simulink model "VirtualVehicleTemplate"  (R2023a)
settings: configuration reference "VehicleVariable" (kept outside this file)
StartFcn:
  | %tic
StopFcn:
  | %toc
undefined symbols (not defined in the file): CtrlEcuRevLim, CtrlTcuInitGear, CtrlVcuCltch1InitCmd, Disabled, DriverPreviewDist, EnvAbsPrs, EnvAirTemp, EnvGrvty, EnvNomFrictionScaling, EnvNominalGrade, EnvWindVelX, EnvWindVelY, EnvWindVelZ, FTP75, PlntVehDstCGFrntAxl, PlntVehDstCGRearAxl, PlntVehInitLatPos, PlntVehInitLongPos, PlntVehInitPitchAng, PlntVehInitRollAng, PlntVehInitVertPos, PlntVehInitYawAng, PlntVehMass, PlntVehTrckWdth, PlntVehYawMomentInertia, ScnCRMaxLatAccel, ScnCRRadius, ScnDLCGateLongPos, ScnDLCLatRef, ScnDLCLatRefOffset, ScnDLCLongRefBpt, ScnDLCLongRefStartPos, ScnDLCVehicleWidth, ScnFHCounterDwellTime, ScnFHInitialDwellTime, ScnFHReturnTime, ScnFHRollRateZeroCross, ScnFHSteerAmp, ScnFHSteerSpeed, ScnISHandwheelRate, ScnISMaxHandwheelAng, ScnISMaxLatAccel, ScnISSteerHoldTime, ScnLongVelRef, ScnSDDwellTime, ScnSDSteerAmp, ScnSDSteerFreq, ScnSimTime, ScnSSFinalFreq, ScnSSSteerAmp, ScnSSSweepTime, ScnStartTime
libraries: simulink x18, vehdynlibscenariocommon x7, vehdynlibviscommon x3, vehdynlibdriver x2, sim3dgroundtruthsensorlib x2, autolibshared x2, autolibsharedcommon x1, sharedtransform x1, sim3dlib x1, sim3dautolib x1
(part 5 of 5)

== system VirtualVehicleTemplate/Environment/Ground Feedback/3D Engine/3D Engine Source/Single Point ==
  Bus Creator1 : BusCreator  Inputs=4
  Bus Selector2 : BusSelector  OutputSignals=Wheel1Positions,Wheel2Positions,Wheel3Positions,Wheel4Positions
  Constant2 : Constant  Value=repmat(eye(3),1,1,4)  SampleTime=-1
  Data Type Conversion{1..4} (4 alike) : DataTypeConversion  SaturateOnIntegerOverflow=off  RndMeth=Floor
  First Order Hold{5..8} (4 alike) : FirstOrderHold  ErrorTolerance=1
  Range Limiter{5..8} (4 alike) : Saturate  UpperLimit=1e3  LowerLimit=-1e3  ZeroCross=off
  Signal Specification{6..9} (4 alike) : SignalSpecification  Unit=m
  Simulation 3D Terrain Sensor1 : sim3dgroundtruthsensorlib/Simulation 3D Terrain Sensor  Priority=1  sensorTag=Sim3dSensor1  sensorId=1  sensorName=Sim3dSensor1  VehicleIdentifier=SimulinkVehicle1  tmountOffset=[0, 0, 0]  rmountOffset=[0,0,0,]  RayOrigins=[0 0 1]  RayDirections=[0 0 -1]  RayLengths=20  NumberOfWheels=4  VisualizeTraceLines=off  SampleTime=-1  aMode=2  ID=1
  Zend Select{1..4} (4 alike) : Selector  NumberOfDimensions=2  InputPortWidth=3  IndexOptions=Select all,Index vector (dialog)  Indices=[1 3],3  OutputSizes=1,1
  z : Outport
  DCM : Outport  Port=2
  wires:
  Signal Specification6/1 -> Bus Creator1/1  "G_FL_z"
  Simulation 3D Terrain Sensor1/1 -> Bus Selector2/1
  Bus Selector2/4 -> Range Limiter8/1  "<Wheel4Positions>"
  Zend Select1/1 -> Data Type Conversion1/1
  Signal Specification7/1 -> Bus Creator1/2  "G_FR_z"
  Bus Selector2/2 -> Range Limiter6/1  "<Wheel2Positions>"
  Data Type Conversion3/1 -> First Order Hold7/1
  Data Type Conversion4/1 -> First Order Hold8/1
  Zend Select3/1 -> Data Type Conversion3/1
  First Order Hold6/1 -> Signal Specification7/1
  Zend Select2/1 -> Data Type Conversion2/1
  Data Type Conversion2/1 -> First Order Hold6/1
  Range Limiter6/1 -> Zend Select2/1
  Data Type Conversion1/1 -> First Order Hold5/1
  First Order Hold7/1 -> Signal Specification8/1
  Zend Select4/1 -> Data Type Conversion4/1
  Range Limiter8/1 -> Zend Select4/1
  Bus Selector2/1 -> Range Limiter5/1  "<Wheel1Positions>"
  First Order Hold8/1 -> Signal Specification9/1
  Bus Selector2/3 -> Range Limiter7/1  "<Wheel3Positions>"
  Range Limiter7/1 -> Zend Select3/1
  First Order Hold5/1 -> Signal Specification6/1
  Range Limiter5/1 -> Zend Select1/1
  Signal Specification8/1 -> Bus Creator1/3  "G_RL_z"
  Signal Specification9/1 -> Bus Creator1/4  "G_RR_z"
  Bus Creator1/1 -> z/1  "z"
  Constant2/1 -> DCM/1  "DCM"

== system VirtualVehicleTemplate/Environment/Varying Friction/Varying Friction/Road Track Friction/2D Lookup Tbl for Scaling Fctr (Lambda) ==
  XWhl : Inport  Partition=on  PartitionDimension=1  PartitionWidth=1  PartitionOffset=0
  YWhl : Inport  Port=2  Partition=on  PartitionDimension=1  PartitionWidth=1  PartitionOffset=0
  XBpt : Inport  Port=3
  YBpt : Inport  Port=4
  2-D Lookup Table : Lookup_n-D  BreakpointsForDimension1Source=Input port  BreakpointsForDimension1=xbr  BreakpointsForDimension2Source=Input port  BreakpointsForDimension2=ybr  Table=mutable  ExtrapMethod=Clip  InternalRulePriority=Speed  RndMeth=Simplest
      settings: InputPortMap=u0,u1,p5,p7
  For Each : ForEach  DisableCoverage=on
  Lambda for each whl : Outport  ConcatenationDimension=1
  wires:
  XWhl/1 -> 2-D Lookup Table/1
  YWhl/1 -> 2-D Lookup Table/2
  2-D Lookup Table/1 -> Lambda for each whl/1
  XBpt/1 -> 2-D Lookup Table/3
  YBpt/1 -> 2-D Lookup Table/4

== system VirtualVehicleTemplate/Environment/Varying Friction/Varying Friction/Road Track Friction/Creating Inertial Frm Bpt ==
  XCg : Inport
  YCg : Inport  Port=2
  Enable : EnablePort
  Add : Sum
  Add1 : Sum
  Constant1 : Constant  Value=ybr
  Constant3 : Constant  Value=xbr
  XBpt : Outport
  YBpt : Outport  Port=2
  wires:
  Add/1 -> XBpt/1
  Constant1/1 -> Add1/1
  Add1/1 -> YBpt/1
  Constant3/1 -> Add/2
  YCg/1 -> Add1/2
  XCg/1 -> Add/1

== system VirtualVehicleTemplate/Environment/Varying Friction/Varying Friction/Road Track Friction/En at t = 0 ==
  Clock1 : Clock
  Compare To Zero : simulink/Logic and Bit Operations/Compare To Zero  relop===  OutDataTypeStr=boolean
  Constant : Constant
  Constant2 : Constant  Value=0
  Switch1 : Switch  Criteria=u2 > Threshold  SaturateOnIntegerOverflow=off  InputSameDT=off
  Out1 : Outport
  wires:
  Clock1/1 -> Compare To Zero/1
  Constant2/1 -> Switch1/3
  Constant/1 -> Switch1/1
  Switch1/1 -> Out1/1
  Compare To Zero/1 -> Switch1/2

== system VirtualVehicleTemplate/Scenarios/Reference Generator/3D Engine/3D Engine/Part Rotation Concatenation ==
  Body Roll : Inport
  Body Ptich : Inport  Port=2
  Body Yaw : Inport  Port=3
  WheelFrontLeft Pitch : Inport  Port=4
  WheelFrontRight Pitch : Inport  Port=5
  WheelRearLeft Pitch : Inport  Port=6
  WheelRearRight Ptich : Inport  Port=7
  WheelFrontLeft Roll : Inport  Port=8
  WheelFrontRight Roll : Inport  Port=9
  WheelRearLeft Roll : Inport  Port=10
  WheelRearRight Roll : Inport  Port=11
  WheelFrontLeft Yaw : Inport  Port=12
  WheelFrontRight Yaw : Inport  Port=13
  WheelRearLeft Yaw : Inport  Port=14
  WheelRearRight Yaw : Inport  Port=15
  AllParts : Concatenate  NumInputs=5  Mode=Multidimensional array
  Body : Concatenate  NumInputs=3  Mode=Multidimensional array  ConcatenateDimension=2
  WheelFrontLeft : Concatenate  NumInputs=3  Mode=Multidimensional array  ConcatenateDimension=2
  WheelFrontRight : Concatenate  NumInputs=3  Mode=Multidimensional array  ConcatenateDimension=2
  WheelRearLeft : Concatenate  NumInputs=3  Mode=Multidimensional array  ConcatenateDimension=2
  WheelRearRight : Concatenate  NumInputs=3  Mode=Multidimensional array  ConcatenateDimension=2
  ConcatOut : Outport  VectorParamsAs1DForOutWhenUnconnected=off
  wires:
  WheelRearRight Roll/1 -> WheelRearRight/1
  WheelRearRight Ptich/1 -> WheelRearRight/2
  WheelRearLeft Roll/1 -> WheelRearLeft/1
  WheelRearLeft Pitch/1 -> WheelRearLeft/2
  WheelFrontRight Roll/1 -> WheelFrontRight/1
  WheelFrontRight Pitch/1 -> WheelFrontRight/2
  WheelFrontLeft Roll/1 -> WheelFrontLeft/1
  WheelFrontLeft Pitch/1 -> WheelFrontLeft/2
  Body Roll/1 -> Body/1
  Body Ptich/1 -> Body/2
  WheelFrontRight Yaw/1 -> WheelFrontRight/3
  WheelRearRight/1 -> AllParts/5
  AllParts/1 -> ConcatOut/1
  WheelRearLeft Yaw/1 -> WheelRearLeft/3
  WheelRearRight Yaw/1 -> WheelRearRight/3
  WheelFrontRight/1 -> AllParts/3
  WheelRearLeft/1 -> AllParts/4
  Body/1 -> AllParts/1
  WheelFrontLeft/1 -> AllParts/2
  WheelFrontLeft Yaw/1 -> WheelFrontLeft/3
  Body Yaw/1 -> Body/3

== system VirtualVehicleTemplate/Scenarios/Reference Generator/3D Engine/3D Engine/Part Translation Concatenation ==
  BodyX : Inport
  BodyY : Inport  Port=2
  BodyZ : Inport  Port=3
  WheelFrontLeftX : Inport  Port=4
  WheelFrontRightX : Inport  Port=5
  WheelRearLeftX : Inport  Port=6
  WheelRearRightX : Inport  Port=7
  WheelFrontLeftY : Inport  Port=8
  WheelFrontRightY : Inport  Port=9
  WheelRearLeftY : Inport  Port=10
  WheelRearRightY : Inport  Port=11
  WheelFrontLeftZ : Inport  Port=12
  WheelFrontRightZ : Inport  Port=13
  WheelRearLeftZ : Inport  Port=14
  WheelRearRightZ : Inport  Port=15
  AllParts : Concatenate  NumInputs=5  Mode=Multidimensional array
  Body : Concatenate  NumInputs=3  Mode=Multidimensional array  ConcatenateDimension=2
  WheelFrontLeft : Concatenate  NumInputs=3  Mode=Multidimensional array  ConcatenateDimension=2
  WheelFrontRight : Concatenate  NumInputs=3  Mode=Multidimensional array  ConcatenateDimension=2
  WheelRearLeft : Concatenate  NumInputs=3  Mode=Multidimensional array  ConcatenateDimension=2
  WheelRearRight : Concatenate  NumInputs=3  Mode=Multidimensional array  ConcatenateDimension=2
  ConcatOut : Outport  VectorParamsAs1DForOutWhenUnconnected=off
  wires:
  WheelFrontRightZ/1 -> WheelFrontRight/3
  WheelRearLeftX/1 -> WheelRearLeft/1
  WheelRearRight/1 -> AllParts/5
  WheelRearLeftY/1 -> WheelRearLeft/2
  AllParts/1 -> ConcatOut/1
  WheelRearLeftZ/1 -> WheelRearLeft/3
  WheelRearRightY/1 -> WheelRearRight/2
  WheelFrontRightX/1 -> WheelFrontRight/1
  WheelFrontRightY/1 -> WheelFrontRight/2
  WheelRearRightZ/1 -> WheelRearRight/3
  WheelFrontRight/1 -> AllParts/3
  WheelRearLeft/1 -> AllParts/4
  Body/1 -> AllParts/1
  WheelRearRightX/1 -> WheelRearRight/1
  WheelFrontLeft/1 -> AllParts/2
  BodyY/1 -> Body/2
  WheelFrontLeftY/1 -> WheelFrontLeft/2
  WheelFrontLeftZ/1 -> WheelFrontLeft/3
  WheelFrontLeftX/1 -> WheelFrontLeft/1
  BodyZ/1 -> Body/3
  BodyX/1 -> Body/1

== system VirtualVehicleTemplate/Scenarios/Reference Generator/3D Engine/3D Engine/Scale ==
  Constant{1..12,17,32..33} (15 alike) : Constant  OutDataTypeStr=single
  PartConcatenation : Subsystem
  ScaleOut : Outport  VectorParamsAs1DForOutWhenUnconnected=off
  wires:
  PartConcatenation/1(ConcatOut) -> ScaleOut/1
  Constant12/1 -> PartConcatenation/1(BodyX)
  Constant17/1 -> PartConcatenation/2(BodyY)
  Constant32/1 -> PartConcatenation/3(BodyZ)
  Constant33/1 -> PartConcatenation/4(WheelFrontLeftX)
  Constant1/1 -> PartConcatenation/5(WheelFrontLeftY)
  Constant2/1 -> PartConcatenation/6(WheelFrontLeftZ)
  Constant5/1 -> PartConcatenation/7(WheelFrontRightX)
  Constant3/1 -> PartConcatenation/8(WheelFrontRightY)
  Constant4/1 -> PartConcatenation/9(WheelFrontRightZ)
  Constant8/1 -> PartConcatenation/10(WheelRearLeftX)
  Constant6/1 -> PartConcatenation/11(WheelRearLeftY)
  Constant7/1 -> PartConcatenation/12(WheelRearLeftZ)
  Constant11/1 -> PartConcatenation/13(WheelRearRightX)
  Constant9/1 -> PartConcatenation/14(WheelRearRightY)
  Constant10/1 -> PartConcatenation/15(WheelRearRightZ)

== system VirtualVehicleTemplate/Environment/Ground Feedback/3D Engine/3D Engine Source/Multiple Points/For Each Subsystem ==
  phi,theta,psi : Inport  Partition=on  PartitionDimension=2  PartitionWidth=1  PartitionOffset=0
  For Each : ForEach  DisableCoverage=on
  Rotation Angles to Direction Cosine Matrix1 : sharedtransform/Rotation Angles to Direction Cosine Matrix  rotationOrder=YXZ  aMode=2
  Selector5 : Selector  InputPortWidth=3  IndexOptions=Index vector (dialog)  Indices=[2 1 3]  OutputSizes=1
  WheelDCM : Outport  ConcatenationDimension=3
  wires:
  Selector5/1 -> Rotation Angles to Direction Cosine Matrix1/1
  Rotation Angles to Direction Cosine Matrix1/1 -> WheelDCM/1
  phi,theta,psi/1 -> Selector5/1

== system VirtualVehicleTemplate/Scenarios/Reference Generator/3D Engine/3D Engine/Scale/PartConcatenation ==
  BodyX : Inport
  BodyY : Inport  Port=2
  BodyZ : Inport  Port=3
  WheelFrontLeftX : Inport  Port=4
  WheelFrontLeftY : Inport  Port=5
  WheelFrontLeftZ : Inport  Port=6
  WheelFrontRightX : Inport  Port=7
  WheelFrontRightY : Inport  Port=8
  WheelFrontRightZ : Inport  Port=9
  WheelRearLeftX : Inport  Port=10
  WheelRearLeftY : Inport  Port=11
  WheelRearLeftZ : Inport  Port=12
  WheelRearRightX : Inport  Port=13
  WheelRearRightY : Inport  Port=14
  WheelRearRightZ : Inport  Port=15
  AllParts : Concatenate  NumInputs=5  Mode=Multidimensional array
  Body : Concatenate  NumInputs=3  Mode=Multidimensional array  ConcatenateDimension=2
  WheelFrontLeft : Concatenate  NumInputs=3  Mode=Multidimensional array  ConcatenateDimension=2
  WheelFrontRight : Concatenate  NumInputs=3  Mode=Multidimensional array  ConcatenateDimension=2
  WheelRearLeft : Concatenate  NumInputs=3  Mode=Multidimensional array  ConcatenateDimension=2
  WheelRearRight : Concatenate  NumInputs=3  Mode=Multidimensional array  ConcatenateDimension=2
  ConcatOut : Outport  VectorParamsAs1DForOutWhenUnconnected=off
  wires:
  WheelFrontRightZ/1 -> WheelFrontRight/3
  WheelRearLeftX/1 -> WheelRearLeft/1
  WheelRearRight/1 -> AllParts/5
  WheelRearLeftY/1 -> WheelRearLeft/2
  AllParts/1 -> ConcatOut/1
  WheelRearLeftZ/1 -> WheelRearLeft/3
  WheelRearRightY/1 -> WheelRearRight/2
  WheelFrontRightX/1 -> WheelFrontRight/1
  WheelFrontRightY/1 -> WheelFrontRight/2
  WheelRearRightZ/1 -> WheelRearRight/3
  WheelFrontRight/1 -> AllParts/3
  WheelRearLeft/1 -> AllParts/4
  Body/1 -> AllParts/1
  WheelRearRightX/1 -> WheelRearRight/1
  WheelFrontLeft/1 -> AllParts/2
  BodyY/1 -> Body/2
  WheelFrontLeftY/1 -> WheelFrontLeft/2
  WheelFrontLeftZ/1 -> WheelFrontLeft/3
  WheelFrontLeftX/1 -> WheelFrontLeft/1
  BodyZ/1 -> Body/3
  BodyX/1 -> Body/1
